simulink model "pide0"  (R2019a)
settings: Solver=FixedStepDiscrete  StartTime=0.0  StopTime=10.0  FixedStep=4e-3  RelTol=1e-3
InitFcn:
  | mbd_mpc574x_consistency_checks(bdroot(gcs));
undefined symbols (not defined in the file): LQFP
libraries: mbd_mpc574x_ec_toolbox x7, simulink x1
settings Model: Creator=Oolon Colluphid  LastModifiedBy=Oolon Colluphid
settings DataIOCC: ExternalInput=off  InitialState=off  SaveOutput=off  SignalLogging=off  SaveTime=off
settings OptimizationCC: DefaultParameterBehavior=Inlined  EnhancedBackFolding=on  PassReuseOutputArgsAs=Individual arguments  OptimizeBlockOrder=speed  DifferentSizesBufferReuse=on  OptimizationCustomize=off
settings DebuggingCC: InheritedTsInSrcMsg=none  SingleTaskRateTransMsg=error  ParameterTunabilityLossMsg=error  UnconnectedInputMsg=error  UnconnectedOutputMsg=error  UnconnectedLineMsg=error  UnknownTsInhSupMsg=error
settings HardwareCC: ProdBitPerPointer=32  ProdBitPerSizeT=32  ProdBitPerPtrDiffT=32  ProdLargestAtomicInteger=Long  ProdLargestAtomicFloat=Double  ProdEndianess=BigEndian  ProdWordSize=32  ProdHWDeviceType=Motorola PowerPC
settings SFSimCC: MATLABDynamicMemAlloc=off
settings RTWCC: SystemTargetFile=mbd_mpc574x.tlc  MakeCommand=mbd_mpc574x_make_rtw  TemplateMakefile=mbd_mpc574x.tmf  Description=Model Based Design Toolbox MPC57xx Code Generation Target  GenerateReport=on  IncludeHyperlinkInReport=on  LaunchReport=on  GenerateTraceInfo=on  GenerateTraceReport=on  GenerateTraceReportSl=on  GenerateTraceReportSf=on  GenerateTraceReportEml=on
settings CodeAppCC: ForceParamTrailComments=on  IgnoreCustomStorageClasses=off  OperatorAnnotations=on  SimulinkDataObjDesc=on  SFDataObjDesc=on  InsertBlockDesc=on
settings STFCustomTargetCC: TargetLangStandard=C99 (ISO)  MultiwordLength=256  CombineOutputUpdateFcns=on  ERTCustomFileBanners=on  SupportContinuousTime=off  SupportNonInlinedSFcns=off  RemoveResetFunc=on  MATLABClassNameForMDSCustomization=Simulink.SoftwareTarget.ERTCustomization  GRTInterface=off  SystemTargetFile=mbd_mpc574x.tlc
settings ERTTargetCC: TargetLangStandard=C99 (ISO)  ParMdlRefBuildCompliant=off  CompOptLevelCompliant=off  ConcurrentExecutionCompliant=off  ModelStepFunctionPrototypeControlCompliant=off  CPPClassGenCompliant=off  UseToolchainInfoCompliant=off  InlinedParameterPlacement=NonHierarchical  ERTSrcFileBannerTemplate=mbd_ert_code_template.cgt  ERTHdrFileBannerTemplate=mbd_ert_code_template.cgt  ERTDataSrcFileTemplate=mbd_ert_code_template.cgt  ERTDataHdrFileTemplate=mbd_ert_code_template.cgt  ERTCustomFileTemplate=example_file_process.tlc

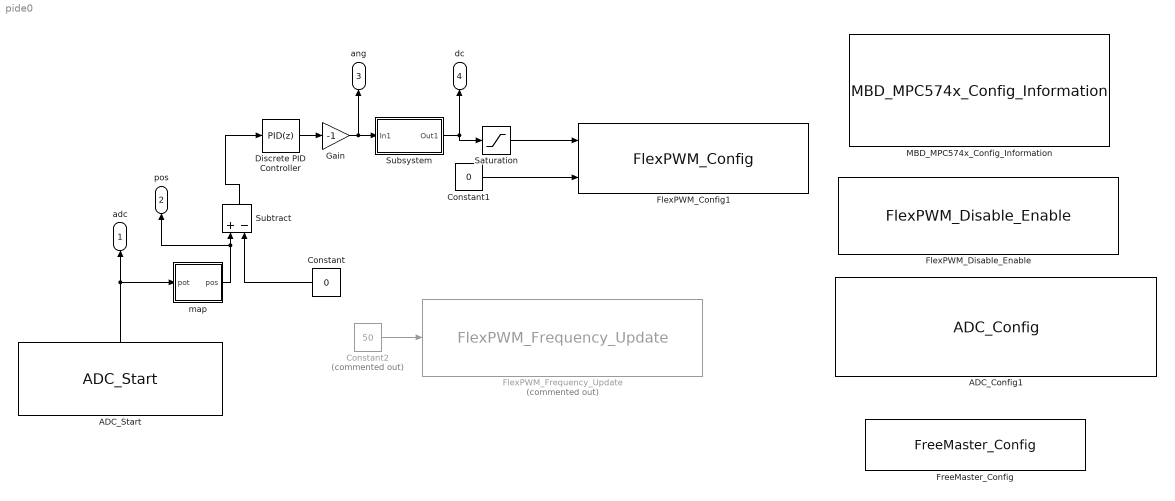
== system pide0 ==
  ADC_Config1 : mbd_mpc574x_ec_toolbox/Motor Control Blocks/ADC Blocks/ADC_Config  adc_instance=1  adc_mode=One-shot  adc_ctu=Disabled  adc_channels_no_n=1  adc_channel_n_0=PTB13: [ADC1_AN0 | Analog function AN0 of ADC1]  adc_channel_n_1=PTB13: [ADC1_AN0 | Analog function AN0 of ADC1]  adc_channel_n_2=PTB13: [ADC1_AN0 | Analog function AN0 of ADC1]  adc_channel_n_3=PTB13: [ADC1_AN0 | Analog function AN0 of ADC1]  adc_channel_n_4=PTB13: [ADC1_AN0 | Analog function AN0 of ADC1]  adc_channel_n_5=PTB13: [ADC1_AN0 | Analog function AN0 of ADC1]  adc_channel_n_6=PTB13: [ADC1_AN0 | Analog function AN0 of ADC1]  adc_channel_n_7=PTB13: [ADC1_AN0 | Analog function AN0 of ADC1]  adc_channel_n_8=PTB13: [ADC1_AN0 | Analog function AN0 of ADC1]  adc_channel_n_9=PTB13: [ADC1_AN0 | Analog function AN0 of ADC1]  adc_channel_n_10=PTB13: [ADC1_AN0 | Analog function AN0 of ADC1]  adc_channel_n_11=PTB13: [ADC1_AN0 | Analog function AN0 of ADC1]  adc_channel_n_12=PTB13: [ADC1_AN0 | Analog function AN0 of ADC1]  show_adv_opts=on  adc_prec=100  adc_presample_0=High voltage ground for ADC  adc_int=100  adc_presample_1=High voltage ground for ADC  adc_ext=100  adc_presample_2=High voltage ground for ADC  adc_clk=Equal to bus clock  adc_ack=off  adc_ext_trigger=External Trigger Disabled  adc_skip_sampling=off  adc_calibration=on  adc_wls=Right  adc_owr=off  adc_inj_trigger=Injected Trigger Disabled  adc_mux_delay=0  adc_decode_delay=0  adc_thr_reg_no=0  adc_upper_value_0=0  adc_lower_value_0=0  adc_upper_value_1=0  adc_lower_value_1=0  adc_upper_value_2=0  adc_lower_value_2=0  adc_upper_value_3=0  adc_lower_value_3=0  adc_upper_value_4=0  adc_lower_value_4=0  adc_upper_value_5=0  adc_lower_value_5=0  adc_upper_value_6=0  adc_lower_value_6=0  adc_upper_value_7=0  adc_lower_value_7=0  adc_upper_value_8=0  adc_lower_value_8=0  adc_upper_value_9=0  adc_lower_value_9=0  adc_upper_value_10=0  adc_lower_value_10=0  adc_upper_value_11=0  adc_lower_value_11=0  adc_upper_value_12=0  adc_lower_value_12=0  adc_upper_value_13=0  adc_lower_value_13=0  adc_upper_value_14=0  adc_lower_value_14=0  adc_upper_value_15=0  adc_lower_value_15=0  adc_wdt_isr_init=off  adc_en_wdt_0=off  adc_th_index_0=0  adc_en_wdt_1=off  adc_th_index_1=0  adc_en_wdt_2=off  adc_th_index_2=0  adc_en_wdt_3=off  adc_th_index_3=0  adc_en_wdt_4=off  adc_th_index_4=0  adc_en_wdt_5=off  adc_th_index_5=0  adc_en_wdt_6=off  adc_th_index_6=0  adc_en_wdt_7=off  adc_th_index_7=0  adc_en_wdt_8=off  adc_th_index_8=0  adc_en_wdt_9=off  adc_th_index_9=0  adc_en_wdt_10=off  adc_th_index_10=0  adc_en_wdt_11=off  adc_th_index_11=0  adc_en_wdt_12=off  adc_th_index_12=0  adc_en_wdt_13=off  adc_th_index_13=0  adc_en_wdt_14=off  adc_th_index_14=0  adc_en_wdt_15=off  adc_th_index_15=0
      settings: SourceProductName=NXP Model-Based Design Toolbox for MPC57xx MCUs
  ADC_Start : mbd_mpc574x_ec_toolbox/Motor Control Blocks/ADC Blocks/ADC_Start  adc_instance=1  interrupt=off  presample=off
      settings: SourceProductName=NXP Model-Based Design Toolbox for MPC57xx MCUs
  Constant : Constant  Value=0  OutDataTypeStr=single
  Constant1 : Constant  Value=0  OutDataTypeStr=single
  Constant2 : Constant  Commented=on  Value=50  OutDataTypeStr=uint32
  Discrete PID Controller : simulink/Continuous/PID Controller  Controller=PID  Form=Parallel  TimeDomain=Discrete-time  SampleTime=4e-3  IntegratorMethod=Forward Euler  FilterMethod=Forward Euler  ControllerParametersSource=internal  P=0.5  I=0.05  D=0.1  UseFilter=on  N=100  TunerSelectOption=Transfer Function Based (PID Tuner App)  InitialConditionSource=internal  InitialConditionForIntegrator=0  InitialConditionForFilter=0  DifferentiatorICPrevScaledInput=0  ExternalReset=none  TrackingMode=off  Kt=1  LimitOutput=on  UpperSaturationLimit=45  LowerSaturationLimit=-45  LinearizeAsGain=off  AntiWindupMode=none  Kb=1  POutMin=[]  POutMax=[]  IOutMin=[]  IOutMax=[]  DOutMin=[]  DOutMax=[]  NOutMin=[]  NOutMax=[]  SumOutMin=[]  SumOutMax=[]  SaturationOutMin=[]  SaturationOutMax=[]  PParamMin=[]  PParamMax=[]  IParamMin=[]  IParamMax=[]  DParamMin=[]  DParamMax=[]  NParamMin=[]  NParamMax=[]  KbParamMin=[]  KbParamMax=[]  KtParamMin=[]  KtParamMax=[]  KbOutMin=[]  KbOutMax=[]  KtOutMin=[]  KtOutMax=[]  IntegratorOutMin=[]  IntegratorOutMax=[]  FilterOutMin=[]  FilterOutMax=[]  SumI1OutMin=[]  SumI1OutMax=[]  SumI2OutMin=[]  SumI2OutMax=[]  SumI3OutMin=[]  SumI3OutMax=[]  SumI4OutMin=[]  SumI4OutMax=[]  SumDOutMin=[]  SumDOutMax=[]  DifferentiatorOutMin=[]  DifferentiatorOutMax=[]  FilterDiffOutCoefMin=[]  FilterDiffOutCoefMax=[]  ReciprocalOutMin=[]  ReciprocalOutMax=[]  SumDenOutMin=[]  SumDenOutMax=[]  SumNumOutMin=[]  SumNumOutMax=[]  DivideOutMin=[]  DivideOutMax=[]  IntegratorContinuousStateAttributes=''  IntegratorStateMustResolveToSignalObject=off  IntegratorRTWStateStorageClass=Auto  FilterContinuousStateAttributes=''  FilterStateMustResolveToSignalObject=off  FilterRTWStateStorageClass=Auto  ParallelPVariant=InternalParameters  IdealPVariant=Disabled  IVariant=InternalParameters  DVariant=InternalParameters  IntegratorVariant=Discrete  SatVariant=Enabled  AWVariant=Passthrough  PCopyVariant=Disabled  TRVariant=Disabled  FdbkBlocksVariant=Forward  IdealPFdbkVariant=Disabled  SatFdbkVariant=Disabled  DerivativeFilterVariant=ForwardEulerFilter  NVariant=InternalParameters  NCopyVariant=Disabled  FilterICVariant=InternalICsFilter  IntegratorICVariant=InternalICs  ExternalResetVariant=Disabled  TRSumVariant=Passthrough  SumFdbkVariant=Disabled  SumVariant=Sum_PID
  FlexPWM_Config1 : mbd_mpc574x_ec_toolbox/Motor Control Blocks/FlexPWM Blocks/FlexPWM_Config  Priority=1  pwmModule=0  pwmSubmodule=0  pwmMode=Edge aligned PWM  pwmPair=Independent  pwmCompSource=PWM23  pwmCounterInit=Local sync (PWMX)  pwmClockSource=Peripheral clock  pwmUnits=Hz  pwmFrequency=50  pwmPeriod=25000  pwmPrescaler=Divide by 64  pwmDtUnits=Nanoseconds  pwmDtNs=50  pwmDtTicks=4  pwmReloadLogic=Full Cycle  pwmReloadFrequency=Every 1 PWM opportunity  pwmTriggeringSignal=Local force signal  pwmDutyCycleOutSim=off  pwmStartAfterInit=on  pwmShowAdvOpts=off  pwmPinA=PTA11: [PWM0_A0 | FlexPWM_0 Channel A Input/Output 0]  pwmPinB=PTA10: [PWM0_B0 | FlexPWM_0 Channel B Input/Output 0]  pwmPolarityA=off  pwmPolarityB=off  pwmAInitialVal=0.075  pwmBInitialVal=0.075  pwmAShift=0  pwmBShift=0  trgReloadISR=off  trgVal0=off  trgVal1=off  trgVal2=off  trgVal3=off  trgVal4=off  trgVal5=off  trgReloadErrorISR=off  pwmPinFault=None  PwmFaultEnISR=off  pwmFaultEnA=off  pwmFaultEnB=off
      settings: SourceProductName=NXP Model-Based Design Toolbox for MPC57xx MCUs
  FlexPWM_Disable_Enable : mbd_mpc574x_ec_toolbox/Motor Control Blocks/FlexPWM Blocks/FlexPWM_Disable_Enable  Priority=1  pwmModule=0  pwmSubmodule0=on  pwmSubmodule1=off  pwmSubmodule2=off  pwmSubmodule3=off  action=Enable
      settings: SourceProductName=NXP Model-Based Design Toolbox for MPC57xx MCUs
  FlexPWM_Frequency_Update : mbd_mpc574x_ec_toolbox/Motor Control Blocks/FlexPWM Blocks/FlexPWM_Frequency_Update  Priority=1  Commented=on  pwmModule=0  pwmSubmodule0=on  pwmSubmodule1=off  pwmSubmodule2=off  pwmSubmodule3=off  pwmUnits=Hz
      settings: SourceProductName=NXP Model-Based Design Toolbox for MPC57xx MCUs
  FreeMaster_Config : mbd_mpc574x_ec_toolbox/Utility Blocks/FreeMaster_Config  interface=Serial1  baudrate=115200  rxd=PTD12: [LIN1_RX | LIN 1 Receive Pin]  txd=PTF14: [LIN1_TX | LINFlexD 1 Transmit Pin]  mode=Short Interrupt  isr_prio=15  show_adv_opts=on  use_scope=on  max_scope_vars=8  use_recorder=on  max_rec_vars=8  rec_buff_size=1024  rec_timebase=0 seconds  comm_buffer_size_auto=on  comm_buffer_size=255  comm_rqueue_size_default=on  comm_rqueue_size=32
      settings: SourceProductName=NXP Model-Based Design Toolbox for MPC57xx MCUs
  Gain : Gain  Gain=-1
  MBD_MPC574x_Config_Information : mbd_mpc574x_ec_toolbox/MBD_MPC574x_Config_Information  disp_str=|  config_params=[]  mcu_target_name=MPC5744P  mcu_target_package=144-LQFP  mcu_target_sram_size=384KB  mcu_system_clock_freq=200  mcu_xtal_freq=40  mcu_step_timer=PIT Channel 0  mcu_step_priority=10  ds_import_enable=on  target_compiler=S32 Design Studio  target_memory=FLASH  s32ds_target_compile_opts=-g3 -mbig -mvle -O1 -mregnames -mlsp -specs=ewl_c9x.specs -mhard-float -Wall -c -std=c99 -fdata-sections -ffunction-sections -funsigned-char -fmessage-length=0 -nostdinc -fno-jump-tables -DTURN_ON_CPU0  s32ds_target_assemble_opts=-g3 -mbig -mvle -mregnames -O1 -DTURN_ON_CPU0 -mhard-float  s32ds_target_link_opts=-Xlinker -gc-sections  s32ds_target_default_lcf=on  s32ds_target_user_lcf=MPC5744P_flash.ld  ghs_target_compile_opts=-preprocess_assembly_files -g -dwarf2 -noSPE -filetype.c  ghs_target_assemble_opts=-preprocess_assembly_files -g -dwarf2 -e _start_core -srec -filetype.assembly  ghs_target_default_lcf=on  ghs_target_user_lcf=MPC5744P_flash.ld  diab_target_compile_opts=-@E+err.log -c -g -Xenum-is-best -Xlint -Xnested-interrupts -Xdebug-local-cie -Xclib-optim-off -Xc-new  diab_target_assemble_opts=-@E+err.log -l -g  diab_target_link_opts=-@E+err.log -Ws -m6 -lc -lm  diab_target_default_lcf=on  diab_target_user_lcf=MPC5744P_flash.dld  pil_download_enable=off  rbl_download_enable=on  rbl_start_delay=5000  rbl_restart_request=on  rbl_com_port=COM9  rbl_com_port_custom=COM6  pil_download_rate=115200  pil_interface=Serial 0  pil_rx=PTB3: [LIN0_RX | LIN 0 Receive Pin]  pil_tx=PTB2: [LIN0_TX | LINFlexD 0 Transmit Pin]  rbl_def_password=on  rbl_password=0xFEEDFACECAFEBEEF  rbl_manual_len_size=off  rbl_start_address=0  rbl_code_size=0  ADC_PcrCheckEnDis=on  FlexPWM_PcrCheckEnDis=on  CTU_PcrCheckEnDis=on  SWG_PcrCheckEnDis=on  eTimer_PcrCheckEnDis=on  FlexCAN_PcrCheckEnDis=on  SPI_PcrCheckEnDis=on  UART_PcrCheckEnDis=on  I2C_PcrCheckEnDis=on  GPIO_OutputPcrCheckEnDis=on  GPIO_InputPcrCheckEnDis=on  eDMA_PcrCheckEnDis=on  PIT_PcrCheckEnDis=on  AMMCLIB_PcrCheckEnDis=on  FM_PcrCheckEnDis=on  Profiler_PcrCheckEnDis=on  ModelRef_PcrCheckEnDis=on  ModelPinCheck_PcrCheckEnDis=on
      | System Clock : 200 MHz
      | Target : MPC5744P
      | Package : 144LQFP
      | XTAL Freq : 40 MHz
      | Compiler : S32 Design Studio
      | Target Type : FLASH
      | Global Interrupt Priority : 8
      | System Tick Interrupt Priority : 12
      | Freemaster : None;
      | Download Code after build : off
      settings: SourceProductName=NXP Model-Based Design Toolbox for MPC57xx MCUs
  Saturation : Saturate  UpperLimit=0.08  LowerLimit=0.06
  Subsystem : Subsystem
  Subtract : Sum  Inputs=+-
  map : Subsystem
  adc : Outport
  pos : Outport  Port=2
  ang : Outport  Port=3
  dc : Outport  Port=4
  wires:
  ADC_Start/1 -> adc/1, map/1(pot)
  Subtract/1 -> Discrete PID Controller/1
  Constant/1 -> Subtract/2
  map/1(pos) -> pos/1, Subtract/1
  Constant2/1 -> FlexPWM_Frequency_Update/1
  Subsystem/1(Out1) -> Saturation/1, dc/1
  Saturation/1 -> FlexPWM_Config1/1
  Constant1/1 -> FlexPWM_Config1/2
  Discrete PID Controller/1 -> Gain/1
  Gain/1 -> Subsystem/1(In1), ang/1

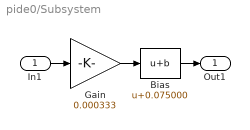
== system pide0/Subsystem ==
  In1 : Inport
  Bias : Bias  Bias=0.075000
  Gain : Gain  Gain=0.000333  OutDataTypeStr=single
  Out1 : Outport
  wires:
  Bias/1 -> Out1/1
  Gain/1 -> Bias/1
  In1/1 -> Gain/1

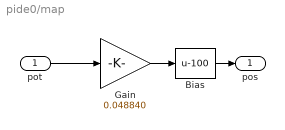
== system pide0/map ==
  pot : Inport
  Bias : Bias  Bias=-100
  Gain : Gain  Gain=0.048840  OutDataTypeStr=single
  pos : Outport
  wires:
  Gain/1 -> Bias/1
  pot/1 -> Gain/1
  Bias/1 -> pos/1
